simulink model "A_ZH_Z4"  (R2025a)
settings: Solver=VariableStepAuto  StartTime=0.0  StopTime=10  RelTol=1e-3
settings Model: Creator=Szalay  LastModifiedBy=Szalay

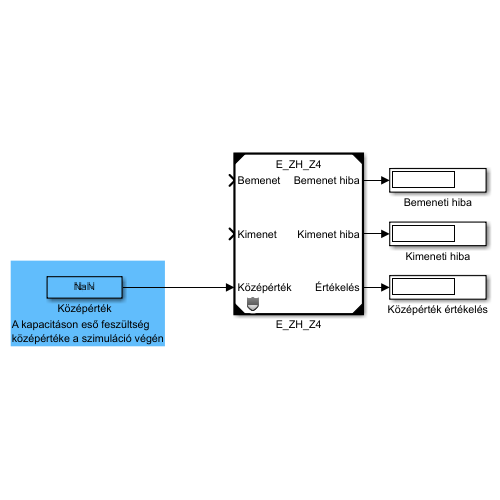
[thumbnail: Simulink's stored preview of the top-level diagram]
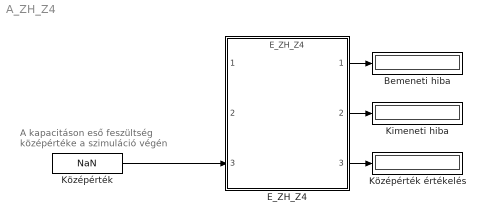
== system A_ZH_Z4 ==
  note: A kapacitáson eső feszültség
      | középértéke a szimuláció végén
  Bemeneti hiba : Display
  E_ZH_Z4 : ModelReference  ModelNameDialog=E_ZH_Z4.slxp  ModelReferenceVersion=1.10  CopyOfModelProtected=on
  Kimeneti hiba : Display
  Középérték : Constant  Value=NaN
  Középérték értékelés : Display
  wires:
  Középérték/1 -> E_ZH_Z4/3
  E_ZH_Z4/3 -> Középérték értékelés/1
  E_ZH_Z4/2 -> Kimeneti hiba/1
  E_ZH_Z4/1 -> Bemeneti hiba/1
